simulink subsystem "Actuator_Manual_Cmd"  (R2025a)
settings: Solver=VariableStepAuto  StartTime=0.0  StopTime=10.0  RelTol=1e-3
settings Model: Creator=gurt1  LastModifiedBy=gurt1

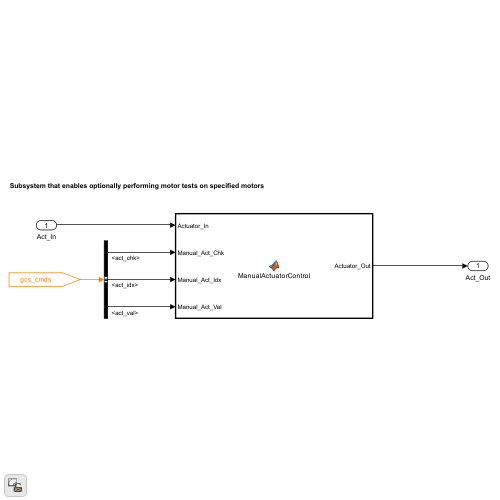
[thumbnail: Simulink's stored preview of the top-level diagram]
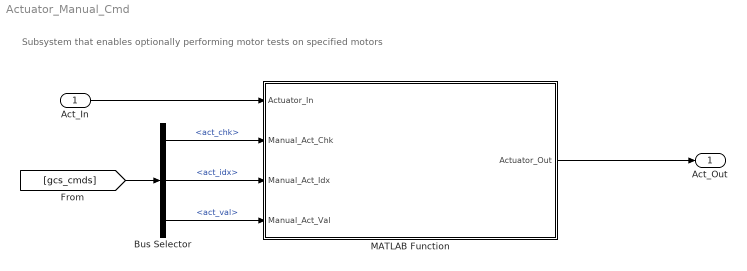
== system Actuator_Manual_Cmd ==
  note: Subsystem that enables optionally performing motor tests on specified motors
  Act_In : Inport
  Bus Selector : BusSelector  OutputSignals=ManualTest.act_chk,ManualTest.act_idx,ManualTest.act_val
  MATLAB Function : MATLAB Function  TreatAsAtomicUnit=on
  Act_Out : Outport
  wires:
  Act_In/1 -> MATLAB Function/1(Actuator_In)
  MATLAB Function/1(Actuator_Out) -> Act_Out/1
  [gcs_cmds] -> Bus Selector/1
  Bus Selector/1 -> MATLAB Function/2(Manual_Act_Chk)  "<act_chk>"
  Bus Selector/2 -> MATLAB Function/3(Manual_Act_Idx)  "<act_idx>"
  Bus Selector/3 -> MATLAB Function/4(Manual_Act_Val)  "<act_val>"

== matlab function Actuator_Manual_Cmd/MATLAB Function ==
  data: Actuator_In input; Actuator_Out output; Manual_Act_Chk input; Manual_Act_Idx input; Manual_Act_Val input
%% ManualActuatorControl
% DESCRIPTION: 
%   This function takes in a 16x1 vector of motor and servo commands and allows 
%   for manual override of individual actuators based on a check parameter. 
%   If the check parameter is set to 1, the value of a specific actuator can be 
%   manually assigned, while the rest will remain at default values.
%   If the index is set to 0, the specified value is sent to all actuators.
%
% INPUTS: 
%   Actuator_In     - (16x1) Input vector of motor and servo commands
%   Manual_Act_Chk  - (1x1) 0 or 1 flag to determine if manual override is active
%   Manual_Act_Val  - (1x1) Value to be sent to the manually selected actuator(s)
%   Manual_Act_Idx  - (1x1) Index of the actuator (1 to 16) to be overridden, 
%                      or 0 to send the value to all actuators
%
% OUTPUTS:
%   Actuator_Out    - (16x1) Output vector for motor and servo commands
% 
% WRITTEN BY:
%   Garrett D. Asper
%   Virginia Tech
%   Email: garrettasper@vt.edu
%
% HISTORY:
%   16 SEP 2024 - Created and debugged, GDA
%
% NOMENCLATURE:                                  UNITS:
%   Not Applicable                                  Not Applicable

function Actuator_Out = ManualActuatorControl(Actuator_In, Manual_Act_Chk, Manual_Act_Idx, Manual_Act_Val)

    % Initialize output vector: -1 for motors (1:8), NaN for servos (9:16)
    Manual_Actuator_Out = [-1 * ones(8, 1); NaN * ones(8, 1)];
    
    % Check boundaries for Manual_Act_Val
    if Manual_Act_Val < 0 || Manual_Act_Val > 1
        Manual_Act_Val = 0; % Default to 0 if outside valid range
    end

    % Check if manual override is active
    if Manual_Act_Chk == 1
        % If index is 0, set value for all actuators
        if Manual_Act_Idx == 0
            % Assign the value to all actuators (motors and servos)
            Manual_Actuator_Out(1:8) = Manual_Act_Val;  % Set all motors to the value
            Manual_Actuator_Out(9:16) = Manual_Act_Val; % Set all servos to the value
        else
            % Check boundaries for Manual_Act_Idx
            if Manual_Act_Idx < 1 || Manual_Act_Idx > 16
                Manual_Act_Idx = 1; % Default to 1 if outside valid range
            end
            % Assign the Manual_Act_Val to the specified actuator
            Manual_Actuator_Out(Manual_Act_Idx) = Manual_Act_Val;
        end
        Actuator_Out = Manual_Actuator_Out;
    else
        Actuator_Out = Actuator_In; % Pass through input vector if no manual override
    end
    
end
